simulink model "V1"  (R2025a)
settings: Solver=VariableStepAuto  StartTime=0.0  StopTime=200  FixedStep=0.005  RelTol=1e-3
libraries: cstblocks x11, vrlib x10, slpidlib x9, simulink_extras x8, dspinverses x3, robotcorelib x2, simulink x1
(part 2 of 3)

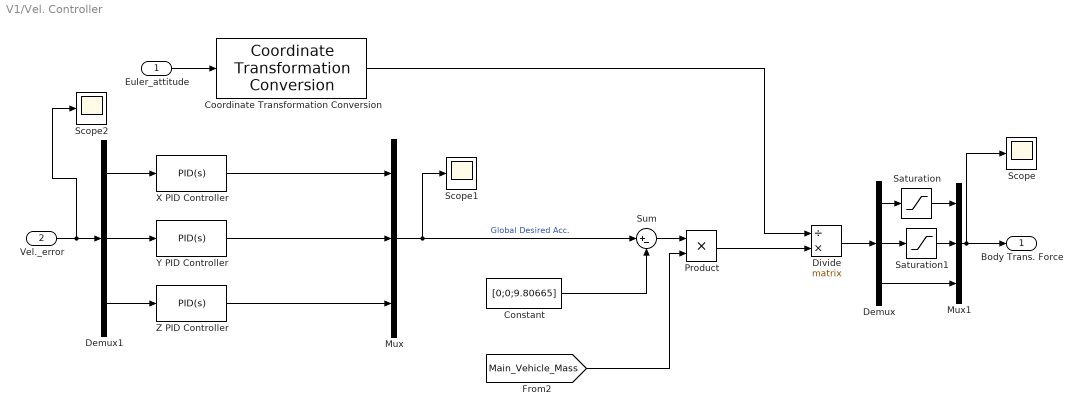
== system V1/Vel. Controller ==
  Euler_attitude : Inport
  Vel._error : Inport  Port=2
  Constant : Constant  Value=[0;0;9.80665]
  Coordinate Transformation Conversion : robotcorelib/Coordinate Transformation Conversion  InputRepresentation=Euler Angles  InputEulerSequence=XYZ  ShowTrVecInputPort=on  OutputRepresentation=Rotation Matrix  OutputEulerSequence=ZYX  ShowTrVecOutputPort=on  SimulateUsing=Interpreted execution
  Demux : Demux  Outputs=3
  Demux1 : Demux  Outputs=3
  Divide : Product  Inputs=/*  Multiplication=Matrix(*)
  Mux : Mux  Inputs=3
  Mux1 : Mux  Inputs=3
  Product : Product
  Saturation : Saturate  UpperLimit=50  LowerLimit=-50
  Saturation1 : Saturate  UpperLimit=50  LowerLimit=-50
  Scope : Scope
      settings: ActiveDisplayYMinimum=-41.94402  ActiveDisplayYMaximum=31.3207  DataLoggingVariableName=ScopeData2
  Scope1 : Scope
      settings: ActiveDisplayYMinimum=-15.22848  ActiveDisplayYMaximum=13.36333
  Scope2 : Scope
      settings: ActiveDisplayYMinimum=-406.2264  ActiveDisplayYMaximum=117.71416  DataLoggingVariableName=ScopeData4
  Sum : Sum  Inputs=|+-
  X PID Controller : slpidlib/PID Controller  Controller=PID  Form=Parallel  TimeDomain=Continuous-time  UseExternalTs=off  SampleTime=-1  IntegratorMethod=Forward Euler  FilterMethod=Forward Euler  ControllerParametersSource=internal  P=3  I=0  UseKiTs=off  D=1  UseExternalDerivativeSource=off  N=100  UseFilter=on  TunerSelectOption=Transfer Function Based (PID Tuner App)  InitialConditionSource=internal  InitialConditionForIntegrator=0  InitialConditionForFilter=0  DifferentiatorICPrevScaledInput=0  ExternalReset=none  TrackingMode=off  Kt=1  LimitOutput=off  SatLimitsSource=internal  UpperSaturationLimit=2  LowerSaturationLimit=-2  LinearizeAsGain=on  AntiWindupMode=none  Kb=1  LimitIntegrator=off  UpperIntegratorSaturationLimit=inf  LowerIntegratorSaturationLimit=-inf  POutMin=[]  POutMax=[]  IOutMin=[]  IOutMax=[]  DOutMin=[]  DOutMax=[]  NOutMin=[]  NOutMax=[]  SumOutMin=[]  SumOutMax=[]  SaturationOutMin=[]  SaturationOutMax=[]  PParamMin=[]  PParamMax=[]  IParamMin=[]  IParamMax=[]  DParamMin=[]  DParamMax=[]  NParamMin=[]  NParamMax=[]  KbParamMin=[]  KbParamMax=[]  KtParamMin=[]  KtParamMax=[]  KbOutMin=[]  KbOutMax=[]  KtOutMin=[]  KtOutMax=[]  IntegratorOutMin=[]  IntegratorOutMax=[]  FilterOutMin=[]  FilterOutMax=[]  SumI1OutMin=[]  SumI1OutMax=[]  SumI2OutMin=[]  SumI2OutMax=[]  SumI3OutMin=[]  SumI3OutMax=[]  SumI4OutMin=[]  SumI4OutMax=[]  SumDOutMin=[]  SumDOutMax=[]  DifferentiatorOutMin=[]  DifferentiatorOutMax=[]  FilterDiffOutCoefMin=[]  FilterDiffOutCoefMax=[]  ReciprocalOutMin=[]  ReciprocalOutMax=[]  SumDenOutMin=[]  SumDenOutMax=[]  SumNumOutMin=[]  SumNumOutMax=[]  DivideOutMin=[]  DivideOutMax=[]  UdiffTsProdOutMin=[]  UdiffTsProdOutMax=[]  NTsProdOutMin=[]  NTsProdOutMax=[]  UintegralTsProdOutMin=[]  UintegralTsProdOutMax=[]  UngainTsProdOutMin=[]  UngainTsProdOutMax=[]  ClampingZeroOutDataTypeStr=Inherit: Inherit via back propagation  ClampingZeroOutMin=[]  ClampingZeroOutMax=[]  FilterDenConstantOutDataTypeStr=Inherit: Inherit via back propagation  FilterDenConstantOutMin=[]  FilterDenConstantOutMax=[]  PCopyOutDataTypeStr=Inherit: Inherit via back propagation  PCopyOutMin=[]  PCopyOutMax=[]  NCopyOutDataTypeStr=Inherit: Inherit via back propagation  NCopyOutMin=[]  NCopyOutMax=[]  IntegratorContinuousStateAttributes=''  IntegratorStateMustResolveToSignalObject=off  IntegratorRTWStateStorageClass=Auto  FilterContinuousStateAttributes=''  FilterStateMustResolveToSignalObject=off  FilterRTWStateStorageClass=Auto  ParallelPVariant=InternalParameters  IdealPVariant=Disabled  IVariant=InternalParameters  DVariant=InternalParameters  IntegratorVariant=Continuous  SatVariant=Disabled  AWVariant=Passthrough  PCopyVariant=Disabled  TRVariant=Disabled  FdbkBlocksVariant=Forward  IdealPFdbkVariant=Disabled  SatFdbkVariant=Disabled  DerivativeFilterVariant=ContFilter  NVariant=InternalParameters  NCopyVariant=Disabled  FilterICVariant=InternalICsFilter  IntegratorICVariant=InternalICs  ExternalResetVariant=Disabled  TRSumVariant=Passthrough  SumFdbkVariant=Disabled  SumVariant=Sum_PID  TsampFilterVariant=InternalTs  TsampNgainVariant=Passthrough  TsampIntegralVariant=Disabled_SignalSpec  ExternalSaturationOutDataTypeStr=Inherit: Same as second input  DerivativeSourceVariant=ErrorSignal  PreIntVariant=InternalPreInt
  Y PID Controller : slpidlib/PID Controller  Controller=PID  Form=Parallel  TimeDomain=Continuous-time  UseExternalTs=off  SampleTime=-1  IntegratorMethod=Forward Euler  FilterMethod=Forward Euler  ControllerParametersSource=internal  P=3  I=0  UseKiTs=off  D=1  UseExternalDerivativeSource=off  N=100  UseFilter=on  TunerSelectOption=Transfer Function Based (PID Tuner App)  InitialConditionSource=internal  InitialConditionForIntegrator=0  InitialConditionForFilter=0  DifferentiatorICPrevScaledInput=0  ExternalReset=none  TrackingMode=off  Kt=1  LimitOutput=off  SatLimitsSource=internal  UpperSaturationLimit=2  LowerSaturationLimit=-2  LinearizeAsGain=on  AntiWindupMode=none  Kb=1  LimitIntegrator=off  UpperIntegratorSaturationLimit=inf  LowerIntegratorSaturationLimit=-inf  POutMin=[]  POutMax=[]  IOutMin=[]  IOutMax=[]  DOutMin=[]  DOutMax=[]  NOutMin=[]  NOutMax=[]  SumOutMin=[]  SumOutMax=[]  SaturationOutMin=[]  SaturationOutMax=[]  PParamMin=[]  PParamMax=[]  IParamMin=[]  IParamMax=[]  DParamMin=[]  DParamMax=[]  NParamMin=[]  NParamMax=[]  KbParamMin=[]  KbParamMax=[]  KtParamMin=[]  KtParamMax=[]  KbOutMin=[]  KbOutMax=[]  KtOutMin=[]  KtOutMax=[]  IntegratorOutMin=[]  IntegratorOutMax=[]  FilterOutMin=[]  FilterOutMax=[]  SumI1OutMin=[]  SumI1OutMax=[]  SumI2OutMin=[]  SumI2OutMax=[]  SumI3OutMin=[]  SumI3OutMax=[]  SumI4OutMin=[]  SumI4OutMax=[]  SumDOutMin=[]  SumDOutMax=[]  DifferentiatorOutMin=[]  DifferentiatorOutMax=[]  FilterDiffOutCoefMin=[]  FilterDiffOutCoefMax=[]  ReciprocalOutMin=[]  ReciprocalOutMax=[]  SumDenOutMin=[]  SumDenOutMax=[]  SumNumOutMin=[]  SumNumOutMax=[]  DivideOutMin=[]  DivideOutMax=[]  UdiffTsProdOutMin=[]  UdiffTsProdOutMax=[]  NTsProdOutMin=[]  NTsProdOutMax=[]  UintegralTsProdOutMin=[]  UintegralTsProdOutMax=[]  UngainTsProdOutMin=[]  UngainTsProdOutMax=[]  ClampingZeroOutDataTypeStr=Inherit: Inherit via back propagation  ClampingZeroOutMin=[]  ClampingZeroOutMax=[]  FilterDenConstantOutDataTypeStr=Inherit: Inherit via back propagation  FilterDenConstantOutMin=[]  FilterDenConstantOutMax=[]  PCopyOutDataTypeStr=Inherit: Inherit via back propagation  PCopyOutMin=[]  PCopyOutMax=[]  NCopyOutDataTypeStr=Inherit: Inherit via back propagation  NCopyOutMin=[]  NCopyOutMax=[]  IntegratorContinuousStateAttributes=''  IntegratorStateMustResolveToSignalObject=off  IntegratorRTWStateStorageClass=Auto  FilterContinuousStateAttributes=''  FilterStateMustResolveToSignalObject=off  FilterRTWStateStorageClass=Auto  ParallelPVariant=InternalParameters  IdealPVariant=Disabled  IVariant=InternalParameters  DVariant=InternalParameters  IntegratorVariant=Continuous  SatVariant=Disabled  AWVariant=Passthrough  PCopyVariant=Disabled  TRVariant=Disabled  FdbkBlocksVariant=Forward  IdealPFdbkVariant=Disabled  SatFdbkVariant=Disabled  DerivativeFilterVariant=ContFilter  NVariant=InternalParameters  NCopyVariant=Disabled  FilterICVariant=InternalICsFilter  IntegratorICVariant=InternalICs  ExternalResetVariant=Disabled  TRSumVariant=Passthrough  SumFdbkVariant=Disabled  SumVariant=Sum_PID  TsampFilterVariant=InternalTs  TsampNgainVariant=Passthrough  TsampIntegralVariant=Disabled_SignalSpec  ExternalSaturationOutDataTypeStr=Inherit: Same as second input  DerivativeSourceVariant=ErrorSignal  PreIntVariant=InternalPreInt
  Z PID Controller : slpidlib/PID Controller  Controller=PID  Form=Parallel  TimeDomain=Continuous-time  UseExternalTs=off  SampleTime=-1  IntegratorMethod=Forward Euler  FilterMethod=Forward Euler  ControllerParametersSource=internal  P=3  I=0  UseKiTs=off  D=1  UseExternalDerivativeSource=off  N=100  UseFilter=on  TunerSelectOption=Transfer Function Based (PID Tuner App)  InitialConditionSource=internal  InitialConditionForIntegrator=0  InitialConditionForFilter=0  DifferentiatorICPrevScaledInput=0  ExternalReset=none  TrackingMode=off  Kt=1  LimitOutput=off  SatLimitsSource=internal  UpperSaturationLimit=3  LowerSaturationLimit=-3  LinearizeAsGain=on  AntiWindupMode=none  Kb=1  LimitIntegrator=off  UpperIntegratorSaturationLimit=inf  LowerIntegratorSaturationLimit=-inf  POutMin=[]  POutMax=[]  IOutMin=[]  IOutMax=[]  DOutMin=[]  DOutMax=[]  NOutMin=[]  NOutMax=[]  SumOutMin=[]  SumOutMax=[]  SaturationOutMin=[]  SaturationOutMax=[]  PParamMin=[]  PParamMax=[]  IParamMin=[]  IParamMax=[]  DParamMin=[]  DParamMax=[]  NParamMin=[]  NParamMax=[]  KbParamMin=[]  KbParamMax=[]  KtParamMin=[]  KtParamMax=[]  KbOutMin=[]  KbOutMax=[]  KtOutMin=[]  KtOutMax=[]  IntegratorOutMin=[]  IntegratorOutMax=[]  FilterOutMin=[]  FilterOutMax=[]  SumI1OutMin=[]  SumI1OutMax=[]  SumI2OutMin=[]  SumI2OutMax=[]  SumI3OutMin=[]  SumI3OutMax=[]  SumI4OutMin=[]  SumI4OutMax=[]  SumDOutMin=[]  SumDOutMax=[]  DifferentiatorOutMin=[]  DifferentiatorOutMax=[]  FilterDiffOutCoefMin=[]  FilterDiffOutCoefMax=[]  ReciprocalOutMin=[]  ReciprocalOutMax=[]  SumDenOutMin=[]  SumDenOutMax=[]  SumNumOutMin=[]  SumNumOutMax=[]  DivideOutMin=[]  DivideOutMax=[]  UdiffTsProdOutMin=[]  UdiffTsProdOutMax=[]  NTsProdOutMin=[]  NTsProdOutMax=[]  UintegralTsProdOutMin=[]  UintegralTsProdOutMax=[]  UngainTsProdOutMin=[]  UngainTsProdOutMax=[]  ClampingZeroOutDataTypeStr=Inherit: Inherit via back propagation  ClampingZeroOutMin=[]  ClampingZeroOutMax=[]  FilterDenConstantOutDataTypeStr=Inherit: Inherit via back propagation  FilterDenConstantOutMin=[]  FilterDenConstantOutMax=[]  PCopyOutDataTypeStr=Inherit: Inherit via back propagation  PCopyOutMin=[]  PCopyOutMax=[]  NCopyOutDataTypeStr=Inherit: Inherit via back propagation  NCopyOutMin=[]  NCopyOutMax=[]  IntegratorContinuousStateAttributes=''  IntegratorStateMustResolveToSignalObject=off  IntegratorRTWStateStorageClass=Auto  FilterContinuousStateAttributes=''  FilterStateMustResolveToSignalObject=off  FilterRTWStateStorageClass=Auto  ParallelPVariant=InternalParameters  IdealPVariant=Disabled  IVariant=InternalParameters  DVariant=InternalParameters  IntegratorVariant=Continuous  SatVariant=Disabled  AWVariant=Passthrough  PCopyVariant=Disabled  TRVariant=Disabled  FdbkBlocksVariant=Forward  IdealPFdbkVariant=Disabled  SatFdbkVariant=Disabled  DerivativeFilterVariant=ContFilter  NVariant=InternalParameters  NCopyVariant=Disabled  FilterICVariant=InternalICsFilter  IntegratorICVariant=InternalICs  ExternalResetVariant=Disabled  TRSumVariant=Passthrough  SumFdbkVariant=Disabled  SumVariant=Sum_PID  TsampFilterVariant=InternalTs  TsampNgainVariant=Passthrough  TsampIntegralVariant=Disabled_SignalSpec  ExternalSaturationOutDataTypeStr=Inherit: Same as second input  DerivativeSourceVariant=ErrorSignal  PreIntVariant=InternalPreInt
  Body Trans. Force : Outport
  wires:
  X PID Controller/1 -> Mux/1
  Demux1/1 -> X PID Controller/1
  Demux1/3 -> Z PID Controller/1
  Demux1/2 -> Y PID Controller/1
  Y PID Controller/1 -> Mux/2
  Mux/1 -> Sum/1, Scope1/1  "Global Desired Acc."
  Z PID Controller/1 -> Mux/3
  Vel._error/1 -> Scope2/1, Demux1/1
  Constant/1 -> Sum/2
  Sum/1 -> Product/1
  Euler_attitude/1 -> Coordinate Transformation Conversion/1
  Coordinate Transformation Conversion/1 -> Divide/1
  [Main_Vehicle_Mass] -> Product/2
  Product/1 -> Divide/2
  Divide/1 -> Demux/1
  Demux/3 -> Mux1/3
  Demux/1 -> Saturation/1
  Demux/2 -> Saturation1/1
  Mux1/1 -> Scope/1, Body Trans. Force/1
  Saturation/1 -> Mux1/1
  Saturation1/1 -> Mux1/2

== system V1/skew-symmetric ==
  In1 : Inport
  Constant16 : Constant  Value=0
  Constant17 : Constant  Value=0
  Constant18 : Constant  Value=0
  Demux2 : Demux  Outputs=3
  Display : Display
  Gain : Gain  Gain=-1
  Gain1 : Gain  Gain=-1
  Gain2 : Gain  Gain=-1
  Mux{13..15,17} (4 alike) : Mux  Inputs=3
  Reshape : Reshape  OutputDimensionality=Customize  OutputDimensions=[3,3]
  Transpose : Math  Operator=transpose
  Out1 : Outport
  wires:
  Constant17/1 -> Mux14/2
  Gain2/1 -> Mux15/1
  Mux13/1 -> Mux17/1
  Reshape/1 -> Transpose/1
  Demux2/3 -> Mux14/1, Gain/1  "fz"
  Demux2/2 -> Gain2/1, Mux13/3  "fy"
  Constant18/1 -> Mux15/3
  Gain1/1 -> Mux14/3
  Demux2/1 -> Mux15/2, Gain1/1  "fx"
  Mux17/1 -> Reshape/1
  Mux14/1 -> Mux17/2
  Transpose/1 -> Display/1, Out1/1
  Mux15/1 -> Mux17/3
  Constant16/1 -> Mux13/1
  Gain/1 -> Mux13/2
  In1/1 -> Demux2/1

== system V1/skew-symmetric1 ==
  Constant16 : Constant  Value=3
  Constant17 : Constant  Value=2
  Constant18 : Constant
  Display : Display
  Mux{13..15,17} (4 alike) : Mux  Inputs=3
  Reshape : Reshape  OutputDimensionality=Customize  OutputDimensions=[3,3]
  Transpose : Math  Operator=transpose
  Out1 : Outport
  wires:
  Constant17/1 -> Mux14/2
  ? -> Mux15/1
  Mux13/1 -> Mux17/1
  Reshape/1 -> Transpose/1
  Constant18/1 -> Mux15/3
  ? -> Mux14/3
  Mux17/1 -> Reshape/1
  Mux14/1 -> Mux17/2
  Transpose/1 -> Display/1, Out1/1
  Mux15/1 -> Mux17/3
  Constant16/1 -> Mux13/1
  ? -> Mux13/2

== system V1/Attitude Controller/Subsystem ==
  Constant : Constant
  M11 : Outport
  wires:
  Constant/1 -> M11/1

== system V1/Attitude Controller/Subsystem1 ==
  Constant : Constant  Value=0
  M12 : Outport
  wires:
  Constant/1 -> M12/1

== system V1/Attitude Controller/Subsystem10 ==
  Product : Product
  Trigonometric Function : Trigonometry  Operator=cos
  Trigonometric Function1 : Trigonometry  Operator=cos
  M33 : Outport
  wires:
  Trigonometric Function/1 -> Product/1
  [roll] -> Trigonometric Function1/1
  [pitch] -> Trigonometric Function/1
  Product/1 -> M33/1
  Trigonometric Function1/1 -> Product/2

== system V1/Attitude Controller/Subsystem2 ==
  Gain : Gain  Gain=-1
  Trigonometric Function : Trigonometry
  M13 : Outport
  wires:
  Trigonometric Function/1 -> Gain/1
  [pitch] -> Trigonometric Function/1
  Gain/1 -> M13/1

== system V1/Attitude Controller/Subsystem4 ==
  Constant : Constant  Value=0
  M21 : Outport
  wires:
  Constant/1 -> M21/1

== system V1/Attitude Controller/Subsystem5 ==
  Trigonometric Function : Trigonometry  Operator=cos
  M22 : Outport
  wires:
  [roll] -> Trigonometric Function/1
  Trigonometric Function/1 -> M22/1

== system V1/Attitude Controller/Subsystem6 ==
  Product : Product
  Trigonometric Function : Trigonometry  Operator=cos
  Trigonometric Function1 : Trigonometry
  M23 : Outport
  wires:
  [pitch] -> Trigonometric Function/1
  Trigonometric Function/1 -> Product/1
  [roll] -> Trigonometric Function1/1
  Trigonometric Function1/1 -> Product/2
  Product/1 -> M23/1

== system V1/Attitude Controller/Subsystem8 ==
  Constant : Constant  Value=0
  M31 : Outport
  wires:
  Constant/1 -> M31/1

== system V1/Attitude Controller/Subsystem9 ==
  Gain : Gain  Gain=-1
  Trigonometric Function : Trigonometry
  M32 : Outport
  wires:
  [roll] -> Trigonometric Function/1
  Trigonometric Function/1 -> Gain/1
  Gain/1 -> M32/1

== system V1/Attitude Controller/Yaw rotation matrix ==
  Demux : Demux  Outputs=3
  Display : Display
  Gain : Gain  Gain=-1
  Mux1 : Mux
  Reshape : Reshape  OutputDimensionality=Customize  OutputDimensions=[2,2]
  Trigonometric Function : Trigonometry  Operator=cos
  Trigonometric Function1 : Trigonometry
  Trigonometric Function2 : Trigonometry
  Trigonometric Function3 : Trigonometry  Operator=cos
  Out1 : Outport
  wires:
  Trigonometric Function3/1 -> Mux1/4
  [current_yaw] -> Trigonometric Function3/1, Trigonometric Function2/1, Trigonometric Function1/1, Trigonometric Function/1
  Trigonometric Function/1 -> Mux1/1
  Reshape/1 -> Out1/1, Display/1
  Mux1/1 -> Reshape/1
  Demux/3 -> [current_yaw]
  [Euler_attitude] -> Demux/1
  Trigonometric Function2/1 -> Gain/1
  Trigonometric Function1/1 -> Mux1/2
  Gain/1 -> Mux1/3

== system V1/Body Frame Torque//Force/Subsystem ==
  theta_1 : Inport
  F1 : Inport  Port=2
  Constant : Constant  Value=sqrt(2)
  Divide : Product  Inputs=*/
  Gain : Gain  Gain=-1
  Mux : Mux  Inputs=3
  Product : Product
  Product2 : Product
  Scope : Scope
      settings: ActiveDisplayYMinimum=-32.89337  ActiveDisplayYMaximum=8.61151  DataLoggingVariableName=ScopeData6
  Trigonometric Function : Trigonometry
  Trigonometric Function2 : Trigonometry  Operator=cos
  F1_vector : Outport
  wires:
  Product/1 -> Divide/1
  F1/1 -> Product/2, Product2/2
  Divide/1 -> Mux/2, Mux/1
  theta_1/1 -> Trigonometric Function2/1, Trigonometric Function/1
  Constant/1 -> Divide/2
  Trigonometric Function2/1 -> Product2/1
  Trigonometric Function/1 -> Product/1
  Product2/1 -> Gain/1
  Gain/1 -> Mux/3
  Mux/1 -> Scope/1, F1_vector/1  "F1_vector"

== system V1/Body Frame Torque//Force/Subsystem1 ==
  theta_2 : Inport
  F2 : Inport  Port=2
  Constant : Constant  Value=sqrt(2)
  Divide : Product  Inputs=*/
  Gain : Gain  Gain=-1
  Gain1 : Gain  Gain=-1
  Mux : Mux  Inputs=3
  Product : Product
  Product2 : Product
  Trigonometric Function : Trigonometry
  Trigonometric Function2 : Trigonometry  Operator=cos
  F2_vector : Outport
  wires:
  Product/1 -> Divide/1
  F2/1 -> Product/2, Product2/2
  Divide/1 -> Gain1/1, Mux/1
  theta_2/1 -> Trigonometric Function2/1, Trigonometric Function/1
  Constant/1 -> Divide/2
  Trigonometric Function2/1 -> Product2/1
  Trigonometric Function/1 -> Product/1
  Product2/1 -> Gain/1
  Gain/1 -> Mux/3
  Mux/1 -> F2_vector/1  "F2_vector"
  Gain1/1 -> Mux/2

== system V1/Body Frame Torque//Force/Subsystem2 ==
  theta_3 : Inport
  F3 : Inport  Port=2
  Constant : Constant  Value=sqrt(2)
  Divide : Product  Inputs=*/
  Gain : Gain  Gain=-1
  Gain1 : Gain  Gain=-1
  Mux : Mux  Inputs=3
  Product : Product
  Product2 : Product
  Trigonometric Function : Trigonometry
  Trigonometric Function2 : Trigonometry  Operator=cos
  F3_vector : Outport
  wires:
  Product/1 -> Divide/1
  F3/1 -> Product/2, Product2/2
  theta_3/1 -> Trigonometric Function2/1, Trigonometric Function/1
  Constant/1 -> Divide/2
  Trigonometric Function2/1 -> Product2/1
  Trigonometric Function/1 -> Product/1
  Product2/1 -> Gain/1
  Gain/1 -> Mux/3
  Mux/1 -> F3_vector/1  "F3_vector"
  Divide/1 -> Gain1/1
  Gain1/1 -> Mux/2, Mux/1

== system V1/Body Frame Torque//Force/Subsystem3 ==
  theta_4 : Inport
  F4 : Inport  Port=2
  Constant : Constant  Value=sqrt(2)
  Divide : Product  Inputs=*/
  Gain : Gain  Gain=-1
  Gain1 : Gain  Gain=-1
  Mux : Mux  Inputs=3
  Product : Product
  Product2 : Product
  Trigonometric Function : Trigonometry
  Trigonometric Function2 : Trigonometry  Operator=cos
  F4_vector : Outport
  wires:
  Product/1 -> Divide/1
  F4/1 -> Product/2, Product2/2
  theta_4/1 -> Trigonometric Function2/1, Trigonometric Function/1
  Constant/1 -> Divide/2
  Trigonometric Function2/1 -> Product2/1
  Trigonometric Function/1 -> Product/1
  Product2/1 -> Gain/1
  Gain/1 -> Mux/3
  Mux/1 -> F4_vector/1  "F4_vector"
  Divide/1 -> Mux/2, Gain1/1
  Gain1/1 -> Mux/1

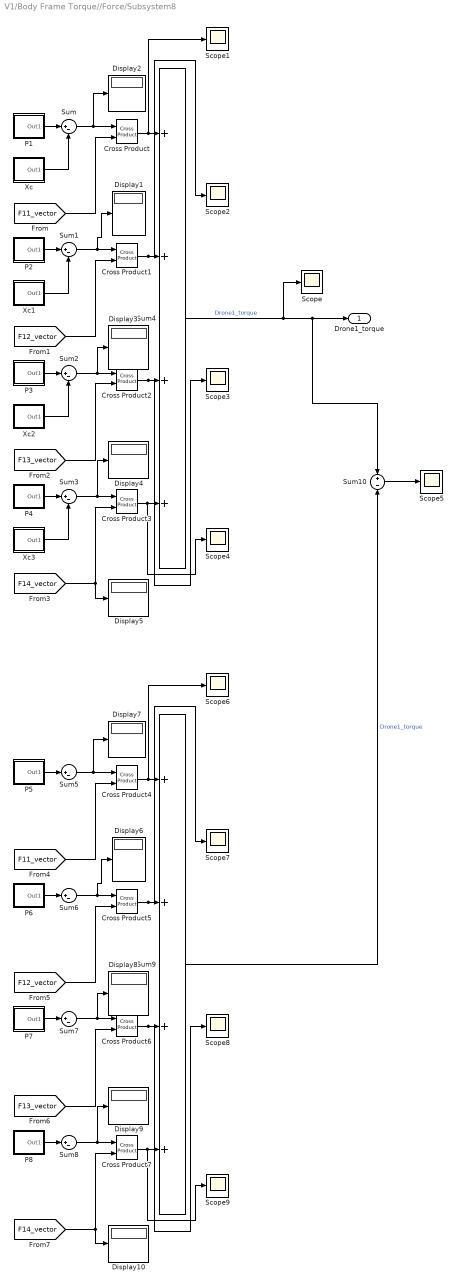
== system V1/Body Frame Torque//Force/Subsystem8 ==
  Cross Product{,1..7} (8 alike) : vrlib/Utilities/Cross Product
  Display{1..10} (10 alike) : Display
  P1 : Subsystem
  P2 : Subsystem
  P3 : Subsystem
  P4 : Subsystem
  P5 : Subsystem
  P6 : Subsystem
  P7 : Subsystem
  P8 : Subsystem
  Scope{,1..9} (10 alike) : Scope
      Scope settings: ActiveDisplayYMinimum=-18.62946  ActiveDisplayYMaximum=66.56889  DataLoggingVariableName=ScopeData4
      Scope1 settings: ActiveDisplayYMinimum=-10.54691  ActiveDisplayYMaximum=29.45294  DataLoggingVariableName=ScopeData10
      Scope2 settings: ActiveDisplayYMinimum=-40.74135  ActiveDisplayYMaximum=40.66911  DataLoggingVariableName=ScopeData11
      Scope3 settings: ActiveDisplayYMinimum=-10.03102  ActiveDisplayYMaximum=8.10812  DataLoggingVariableName=ScopeData15
      Scope4 settings: ActiveDisplayYMinimum=-1.76721  ActiveDisplayYMaximum=9.28155  DataLoggingVariableName=ScopeData16
      Scope5 settings: ActiveDisplayYMinimum=-2.09272  ActiveDisplayYMaximum=0.49282
      Scope6 settings: ActiveDisplayYMinimum=-10.73688  ActiveDisplayYMaximum=29.98451  DataLoggingVariableName=ScopeData2
      Scope7 settings: ActiveDisplayYMinimum=-56.63794  ActiveDisplayYMaximum=56.46415  DataLoggingVariableName=ScopeData3
      Scope8 settings: ActiveDisplayYMinimum=-10.03102  ActiveDisplayYMaximum=8.10812  DataLoggingVariableName=ScopeData4
      Scope9 settings: ActiveDisplayYMinimum=-1.76721  ActiveDisplayYMaximum=9.28155  DataLoggingVariableName=ScopeData5
  Sum{,1..3,5..8} (8 alike) : Sum  Inputs=|+-
  Sum10 : Sum  Inputs=+|-
  Sum4 : Sum  Inputs=++++
  Sum9 : Sum  Inputs=++++
  Xc : Subsystem
  Xc1 : Subsystem
  Xc2 : Subsystem
  Xc3 : Subsystem
  Drone1_torque : Outport
  wires:
  Xc3/1(Out1) -> Sum3/2
  Xc2/1(Out1) -> Sum2/2
  P4/1(Out1) -> Sum3/1
  [F11_vector] -> Cross Product/2
  [F12_vector] -> Cross Product1/2
  P3/1(Out1) -> Sum2/1
  Sum1/1 -> Cross Product1/1, Display1/1
  Cross Product1/1 -> Scope2/1, Sum4/2
  Xc/1(Out1) -> Sum/2
  [F14_vector] -> Cross Product3/2, Display5/1
  Sum/1 -> Display2/1, Cross Product/1
  P1/1(Out1) -> Sum/1
  Cross Product/1 -> Scope1/1, Sum4/1
  Xc1/1(Out1) -> Sum1/2
  Sum3/1 -> Display4/1, Cross Product3/1
  Sum2/1 -> Cross Product2/1, Display3/1
  [F13_vector] -> Cross Product2/2
  Cross Product2/1 -> Scope3/1, Sum4/3
  Cross Product3/1 -> Scope4/1, Sum4/4
  P2/1(Out1) -> Sum1/1
  Sum4/1 -> Scope/1, Sum10/1, Drone1_torque/1  "Drone1_torque"
  P8/1(Out1) -> Sum8/1
  Cross Product4/1 -> Scope6/1, Sum9/1
  Cross Product6/1 -> Scope8/1, Sum9/3
  Sum6/1 -> Cross Product5/1, Display6/1
  P6/1(Out1) -> Sum6/1
  P5/1(Out1) -> Sum5/1
  Cross Product7/1 -> Scope9/1, Sum9/4
  Cross Product5/1 -> Scope7/1, Sum9/2
  Sum5/1 -> Display7/1, Cross Product4/1
  [F13_vector] -> Cross Product6/2
  ? -> Sum5/2
  Sum7/1 -> Cross Product6/1, Display8/1
  [F11_vector] -> Cross Product4/2
  ? -> Sum6/2
  Sum8/1 -> Display9/1, Cross Product7/1
  [F14_vector] -> Cross Product7/2, Display10/1
  [F12_vector] -> Cross Product5/2
  ? -> Sum8/2
  Sum9/1 -> Sum10/2  "Drone1_torque"
  P7/1(Out1) -> Sum7/1
  ? -> Sum7/2
  Sum10/1 -> Scope5/1

== system V1/Non-sequential mixer/Wrench allocation_Drone1 ==
  In1 : Inport
  Bus Selector : BusSelector  OutputSignals=F_x,F_y,F_z
  Bus Selector2 : BusSelector  OutputSignals=tau_x,tau_y,tau_z
  Mux10 : Mux  Inputs=2
  Mux8 : Mux  Inputs=3
  Mux9 : Mux  Inputs=3
  Out1 : Outport
  wires:
  Bus Selector/2 -> Mux8/2  "<F_y>"
  Mux8/1 -> Mux10/2
  In1/1 -> Bus Selector/1, Bus Selector2/1
  Bus Selector2/3 -> Mux9/3  "<tau_z>"
  Bus Selector2/2 -> Mux9/2  "<tau_y>"
  Mux9/1 -> Mux10/1
  Bus Selector2/1 -> Mux9/1  "<tau_x>"
  Mux10/1 -> Out1/1
  Bus Selector/1 -> Mux8/1  "<F_x>"
  Bus Selector/3 -> Mux8/3  "<F_z>"

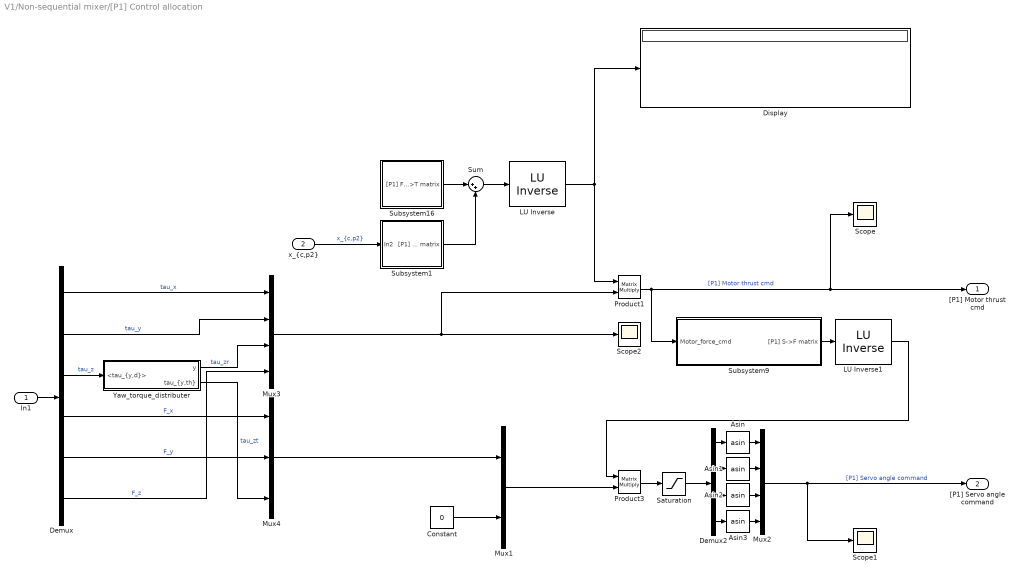
== system V1/Non-sequential mixer/[P1] Control allocation ==
  In1 : Inport
  "x_{c,p2}" : Inport  Port=2
  " LU Inverse" : dspinverses/ LU Inverse
  " LU Inverse1" : dspinverses/ LU Inverse
  Asin{,1..3} (4 alike) : Trigonometry  Operator=asin  OutputSignalType=real
  Constant : Constant  Value=0
  Demux : Demux  Outputs=6
  Demux2 : Demux
  Display : Display
  Mux1 : Mux  Inputs=2
  Mux2 : Mux
  Mux3 : Mux
  Mux4 : Mux  Inputs=3
  Product1 : Product  Multiplication=Matrix(*)
  Product3 : Product  Multiplication=Matrix(*)
  Saturation : Saturate  UpperLimit=0.9  LowerLimit=-0.9
  Scope : Scope
      settings: ActiveDisplayYMinimum=9.1632  ActiveDisplayYMaximum=24.163  DataLoggingVariableName=ScopeData3
  Scope1 : Scope
      settings: ActiveDisplayYMinimum=-1.39971  ActiveDisplayYMaximum=1.39971  DataLoggingVariableName=ScopeData4
  Scope2 : Scope
      settings: ActiveDisplayYMinimum=-7820.2372  ActiveDisplayYMaximum=1813.73582  DataLoggingVariableName=ScopeData5
  Subsystem1 : Subsystem
  Subsystem16 : Subsystem
  Subsystem9 : Subsystem
  Sum : Sum  Inputs=|++
  Yaw_torque_distributer : Subsystem
  "[P1] Motor thrust cmd" : Outport
  "[P1] Servo angle command" : Outport  Port=2
  wires:
  Product3/1 -> Saturation/1
  Subsystem9/1("[P1] S->F matrix") -> " LU Inverse1"/1
  Sum/1 -> " LU Inverse"/1
  Demux2/2 -> Asin1/1
  Asin1/1 -> Mux2/2
  Product1/1 -> Scope/1, "[P1] Motor thrust cmd"/1, Subsystem9/1(Motor_force_cmd)  "[P1] Motor thrust cmd"
  Mux1/1 -> Product3/2
  Asin2/1 -> Mux2/3
  " LU Inverse"/1 -> Product1/1, Display/1
  Mux2/1 -> Scope1/1, "[P1] Servo angle command"/1  "[P1] Servo angle command"
  Asin/1 -> Mux2/1
  Demux2/3 -> Asin2/1
  Asin3/1 -> Mux2/4
  Demux2/1 -> Asin/1
  " LU Inverse1"/1 -> Product3/1
  Demux2/4 -> Asin3/1
  Saturation/1 -> Demux2/1
  In1/1 -> Demux/1
  Demux/3 -> Yaw_torque_distributer/1("<tau_{y,d}>")  "tau_z"
  Demux/1 -> Mux3/1  "tau_x"
  Demux/2 -> Mux3/2  "tau_y"
  Yaw_torque_distributer/1(y) -> Mux3/3  "tau_zr"
  Demux/6 -> Mux3/4  "F_z"
  Demux/4 -> Mux4/1  "F_x"
  Demux/5 -> Mux4/2  "F_y"
  Yaw_torque_distributer/2("tau_{y,th}") -> Mux4/3  "tau_zt"
  "x_{c,p2}"/1 -> Subsystem1/1(In2)  "x_{c,p2}"
  Subsystem16/1("[P1] F->T matrix") -> Sum/1
  Subsystem1/1("[P1] F->T matrix") -> Sum/2
  Mux3/1 -> Scope2/1, Product1/2
  Mux4/1 -> Mux1/1
  Constant/1 -> Mux1/2

== system V1/Body Frame Torque//Force/Subsystem8/P1 ==
  Gain : Gain  Gain=1/sqrt(2)
  Gain1 : Gain  Gain=-1
  Mux : Mux  Inputs=3
  Out1 : Outport
  wires:
  Gain1/1 -> Mux/2
  [a] -> Mux/3
  [l] -> Gain/1
  Gain/1 -> Gain1/1, Mux/1
  Mux/1 -> Out1/1

== system V1/Body Frame Torque//Force/Subsystem8/P2 ==
  Gain : Gain  Gain=1/sqrt(2)
  Gain1 : Gain  Gain=-1
  Gain2 : Gain  Gain=-1
  Mux : Mux  Inputs=3
  Out1 : Outport
  wires:
  Gain1/1 -> Mux/2
  [a] -> Mux/3
  [l] -> Gain/1
  Gain/1 -> Gain1/1, Gain2/1
  Mux/1 -> Out1/1
  Gain2/1 -> Mux/1

== system V1/Body Frame Torque//Force/Subsystem8/P3 ==
  Gain : Gain  Gain=1/sqrt(2)
  Gain1 : Gain  Gain=-1
  Mux : Mux  Inputs=3
  Out1 : Outport
  wires:
  Gain/1 -> Mux/2, Gain1/1
  [a] -> Mux/3
  [l] -> Gain/1
  Mux/1 -> Out1/1
  Gain1/1 -> Mux/1

== system V1/Body Frame Torque//Force/Subsystem8/P4 ==
  Gain : Gain  Gain=1/sqrt(2)
  Mux : Mux  Inputs=3
  Out1 : Outport
  wires:
  Gain/1 -> Mux/2, Mux/1
  [a] -> Mux/3
  [l] -> Gain/1
  Mux/1 -> Out1/1

== system V1/Body Frame Torque//Force/Subsystem8/P5 ==
  Gain : Gain  Gain=1/sqrt(2)
  Gain1 : Gain  Gain=-1
  Mux : Mux  Inputs=3
  Out1 : Outport
  wires:
  Gain1/1 -> Mux/2
  [a] -> Mux/3
  [l] -> Gain/1
  Gain/1 -> Gain1/1, Mux/1
  Mux/1 -> Out1/1

== system V1/Body Frame Torque//Force/Subsystem8/P6 ==
  Gain : Gain  Gain=1/sqrt(2)
  Gain1 : Gain  Gain=-1
  Gain2 : Gain  Gain=-1
  Mux : Mux  Inputs=3
  Out1 : Outport
  wires:
  Gain1/1 -> Mux/2
  [a] -> Mux/3
  [l] -> Gain/1
  Gain/1 -> Gain1/1, Gain2/1
  Mux/1 -> Out1/1
  Gain2/1 -> Mux/1

== system V1/Body Frame Torque//Force/Subsystem8/P7 ==
  Gain : Gain  Gain=1/sqrt(2)
  Gain1 : Gain  Gain=-1
  Mux : Mux  Inputs=3
  Out1 : Outport
  wires:
  Gain/1 -> Mux/2, Gain1/1
  [a] -> Mux/3
  [l] -> Gain/1
  Mux/1 -> Out1/1
  Gain1/1 -> Mux/1

== system V1/Body Frame Torque//Force/Subsystem8/P8 ==
  Gain : Gain  Gain=1/sqrt(2)
  Mux : Mux  Inputs=3
  Out1 : Outport
  wires:
  Gain/1 -> Mux/2, Mux/1
  [a] -> Mux/3
  [l] -> Gain/1
  Mux/1 -> Out1/1

== system V1/Body Frame Torque//Force/Subsystem8/Xc ==
  Mux : Mux  Inputs=3
  Out1 : Outport
  wires:
  [x_c] -> Mux/1
  [z_c] -> Mux/3
  Mux/1 -> Out1/1
  [y_c] -> Mux/2

== system V1/Body Frame Torque//Force/Subsystem8/Xc1 ==
  Mux : Mux  Inputs=3
  Out1 : Outport
  wires:
  [x_c] -> Mux/1
  [z_c] -> Mux/3
  Mux/1 -> Out1/1
  [y_c] -> Mux/2

== system V1/Body Frame Torque//Force/Subsystem8/Xc2 ==
  Mux : Mux  Inputs=3
  Out1 : Outport
  wires:
  [x_c] -> Mux/1
  [z_c] -> Mux/3
  Mux/1 -> Out1/1
  [y_c] -> Mux/2

== system V1/Body Frame Torque//Force/Subsystem8/Xc3 ==
  Mux : Mux  Inputs=3
  Out1 : Outport
  wires:
  [x_c] -> Mux/1
  [z_c] -> Mux/3
  Mux/1 -> Out1/1
  [y_c] -> Mux/2

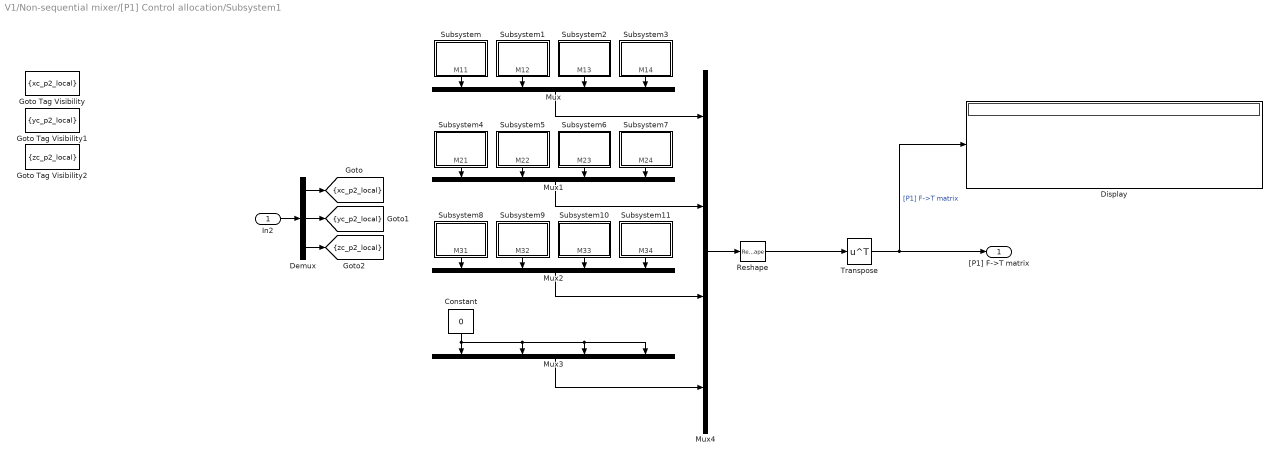
== system V1/Non-sequential mixer/[P1] Control allocation/Subsystem1 ==
  In2 : Inport
  Constant : Constant  Value=0
  Demux : Demux  Outputs=3
  Display : Display
  Goto Tag Visibility : GotoTagVisibility  GotoTag=xc_p2_local
  Goto Tag Visibility1 : GotoTagVisibility  GotoTag=yc_p2_local
  Goto Tag Visibility2 : GotoTagVisibility  GotoTag=zc_p2_local
  Mux{,1..4} (5 alike) : Mux
  Reshape : Reshape  OutputDimensionality=Customize  OutputDimensions=[4,4]
  Subsystem : Subsystem
  Subsystem1 : Subsystem
  Subsystem10 : Subsystem
  Subsystem11 : Subsystem
  Subsystem2 : Subsystem
  Subsystem3 : Subsystem
  Subsystem4 : Subsystem
  Subsystem5 : Subsystem
  Subsystem6 : Subsystem
  Subsystem7 : Subsystem
  Subsystem8 : Subsystem
  Subsystem9 : Subsystem
  Transpose : Math  Operator=transpose
  "[P1] F->T matrix" : Outport
  tag scope: xc_p2_local=scoped, yc_p2_local=scoped, zc_p2_local=scoped
  wires:
  Subsystem2/1(M13) -> Mux/3
  Constant/1 -> Mux3/4, Mux3/3, Mux3/2, Mux3/1
  Mux4/1 -> Reshape/1
  Subsystem8/1(M31) -> Mux2/1
  Mux3/1 -> Mux4/4
  Subsystem1/1(M12) -> Mux/2
  Subsystem5/1(M22) -> Mux1/2
  Subsystem11/1(M34) -> Mux2/4
  Subsystem7/1(M24) -> Mux1/4
  Reshape/1 -> Transpose/1
  Mux/1 -> Mux4/1
  Subsystem10/1(M33) -> Mux2/3
  Mux2/1 -> Mux4/3
  Subsystem3/1(M14) -> Mux/4
  Subsystem4/1(M21) -> Mux1/1
  Subsystem6/1(M23) -> Mux1/3
  Subsystem9/1(M32) -> Mux2/2
  Mux1/1 -> Mux4/2
  Subsystem/1(M11) -> Mux/1
  Transpose/1 -> "[P1] F->T matrix"/1, Display/1  "[P1] F->T matrix"
  In2/1 -> Demux/1
  Demux/1 -> [xc_p2_local]
  Demux/3 -> [zc_p2_local]
  Demux/2 -> [yc_p2_local]

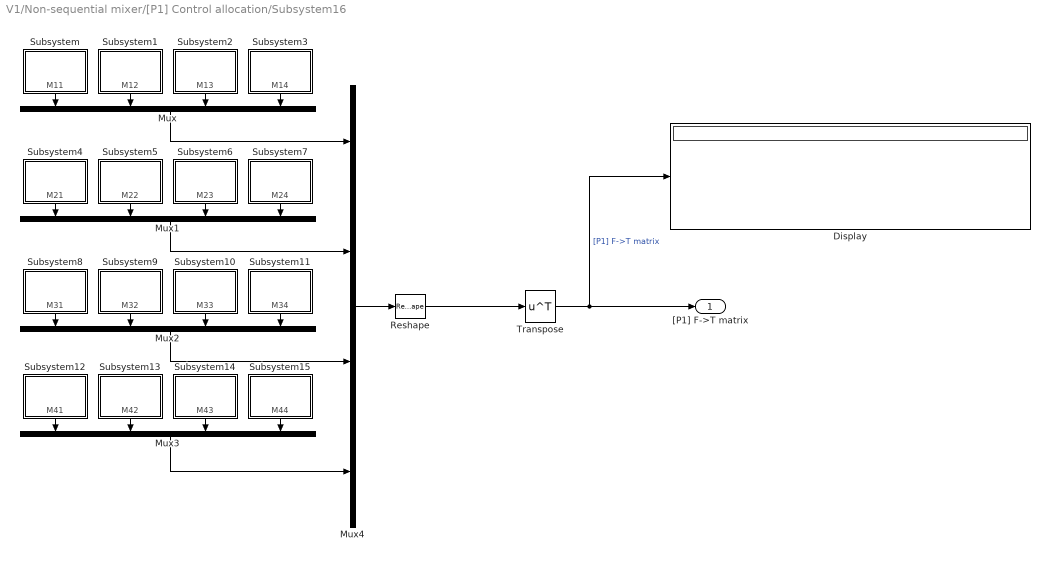
== system V1/Non-sequential mixer/[P1] Control allocation/Subsystem16 ==
  Display : Display
  Mux{,1..4} (5 alike) : Mux
  Reshape : Reshape  OutputDimensionality=Customize  OutputDimensions=[4,4]
  Subsystem : Subsystem
  Subsystem1 : Subsystem
  Subsystem10 : Subsystem
  Subsystem11 : Subsystem
  Subsystem12 : Subsystem
  Subsystem13 : Subsystem
  Subsystem14 : Subsystem
  Subsystem15 : Subsystem
  Subsystem2 : Subsystem
  Subsystem3 : Subsystem
  Subsystem4 : Subsystem
  Subsystem5 : Subsystem
  Subsystem6 : Subsystem
  Subsystem7 : Subsystem
  Subsystem8 : Subsystem
  Subsystem9 : Subsystem
  Transpose : Math  Operator=transpose
  "[P1] F->T matrix" : Outport
  wires:
  Subsystem2/1(M13) -> Mux/3
  Subsystem15/1(M44) -> Mux3/4
  Mux4/1 -> Reshape/1
  Subsystem8/1(M31) -> Mux2/1
  Subsystem14/1(M43) -> Mux3/3
  Mux3/1 -> Mux4/4
  Subsystem1/1(M12) -> Mux/2
  Subsystem5/1(M22) -> Mux1/2
  Subsystem11/1(M34) -> Mux2/4
  Subsystem7/1(M24) -> Mux1/4
  Reshape/1 -> Transpose/1
  Mux/1 -> Mux4/1
  Subsystem10/1(M33) -> Mux2/3
  Mux2/1 -> Mux4/3
  Subsystem3/1(M14) -> Mux/4
  Subsystem12/1(M41) -> Mux3/1
  Subsystem13/1(M42) -> Mux3/2
  Subsystem4/1(M21) -> Mux1/1
  Subsystem6/1(M23) -> Mux1/3
  Subsystem9/1(M32) -> Mux2/2
  Mux1/1 -> Mux4/2
  Subsystem/1(M11) -> Mux/1
  Transpose/1 -> "[P1] F->T matrix"/1, Display/1  "[P1] F->T matrix"

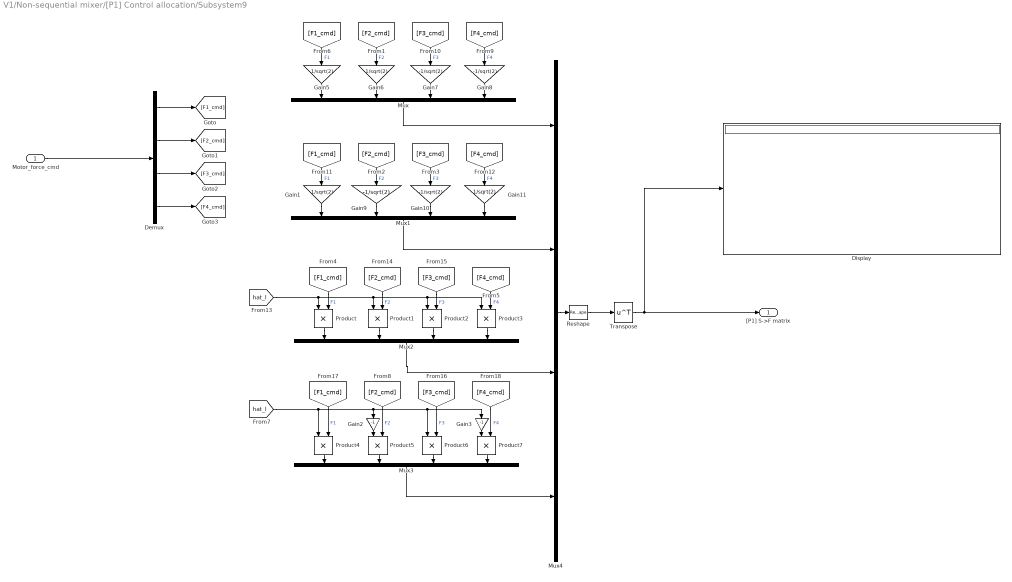
== system V1/Non-sequential mixer/[P1] Control allocation/Subsystem9 ==
  Motor_force_cmd : Inport
  Demux : Demux
  Display : Display
  Gain{1,5..6,11} (4 alike) : Gain  Gain=1/sqrt(2)
  Gain{7..10} (4 alike) : Gain  Gain=-1/sqrt(2)
  Gain2 : Gain  Gain=-1
  Gain3 : Gain  Gain=-1
  Mux{,1..4} (5 alike) : Mux
  Product{,1..7} (8 alike) : Product
  Reshape : Reshape  OutputDimensionality=Customize  OutputDimensions=[4,4]
  Transpose : Math  Operator=transpose
  "[P1] S->F matrix" : Outport
  wires:
  [F2_cmd] -> Gain6/1  "F2"
  Mux/1 -> Mux4/1
  Demux/2 -> [F2_cmd]
  [F1_cmd] -> Gain5/1  "F1"
  Demux/4 -> [F4_cmd]
  Mux3/1 -> Mux4/4
  Demux/3 -> [F3_cmd]
  Mux1/1 -> Mux4/2
  Mux2/1 -> Mux4/3
  Demux/1 -> [F1_cmd]
  Motor_force_cmd/1 -> Demux/1
  Mux4/1 -> Reshape/1
  Reshape/1 -> Transpose/1
  Transpose/1 -> "[P1] S->F matrix"/1, Display/1
  Gain5/1 -> Mux/1
  Gain6/1 -> Mux/2
  [F4_cmd] -> Gain8/1  "F4"
  [F3_cmd] -> Gain7/1  "F3"
  Gain7/1 -> Mux/3
  Gain8/1 -> Mux/4
  Gain9/1 -> Mux1/2
  Gain1/1 -> Mux1/1
  [F1_cmd] -> Gain1/1  "F1"
  [F2_cmd] -> Gain9/1  "F2"
  Gain11/1 -> Mux1/4
  Gain10/1 -> Mux1/3
  [F4_cmd] -> Gain11/1  "F4"
  [F3_cmd] -> Gain10/1  "F3"
  Product/1 -> Mux2/1
  Product1/1 -> Mux2/2
  Product2/1 -> Mux2/3
  Product3/1 -> Mux2/4
  [hat_l] -> Product3/1, Product2/1, Product1/1, Product/1
  [F1_cmd] -> Product/2  "F1"
  [F2_cmd] -> Product1/2  "F2"
  [F3_cmd] -> Product2/2  "F3"
  [F4_cmd] -> Product3/2  "F4"
  [hat_l] -> Gain3/1, Product6/1, Gain2/1, Product4/1
  [F4_cmd] -> Product7/2  "F4"
  Product5/1 -> Mux3/2
  Product4/1 -> Mux3/1
  Product7/1 -> Mux3/4
  [F2_cmd] -> Product5/2  "F2"
  Product6/1 -> Mux3/3
  [F3_cmd] -> Product6/2  "F3"
  [F1_cmd] -> Product4/2  "F1"
  Gain2/1 -> Product5/1
  Gain3/1 -> Product7/1

== system V1/Non-sequential mixer/[P1] Control allocation/Yaw_torque_distributer ==
  "<tau_{y,d}>" : Inport
  Gain : Gain  Gain=-1
  LTI System : cstblocks/LTI System  sys=tf(1,[1 10])  IC=[]  PadeOrder=0
  Saturation Dynamic : simulink/Discontinuities/Saturation Dynamic  OutMin=[]  OutMax=[]  OutDataTypeStr=Inherit: Same as second input  OutDataType=fixdt(1, 16)  OutScaling=2^-10  DoSatur=off
  Scope : Scope  NumInputPorts=2
      settings: ActiveDisplayYMinimum=-0.98774  ActiveDisplayYMaximum=2.13909
  Sum : Sum  Inputs=+-|
  Sum1 : Sum  Inputs=|+-
  Sum2 : Sum  Inputs=++|
  y : Outport
  "tau_{y,th}" : Outport  Port=2
  wires:
  Saturation Dynamic/1 -> Sum/2, Scope/1, y/1
  [yaw_torque_limit] -> Gain/1, Saturation Dynamic/1
  "<tau_{y,d}>"/1 -> Sum1/1, LTI System/1
  Gain/1 -> Saturation Dynamic/3
  LTI System/1 -> Sum1/2, Sum2/2
  Sum1/1 -> Sum/1, Saturation Dynamic/2  "tau_{y,th}"
  Sum/1 -> Sum2/1  "tau_{y,th}"
  Sum2/1 -> Scope/2, "tau_{y,th}"/1  "tau_{y,th}"

== system V1/Non-sequential mixer/[P1] Control allocation/Subsystem1/Subsystem ==
  Bus Selector : BusSelector  OutputSignals=theta_1
  Bus Selector1 : BusSelector  OutputSignals=theta_1
  Gain2 : Gain  Gain=1/sqrt(2)
  Product : Product
  Product1 : Product
  Sum1 : Sum  Inputs=|++
  Trigonometric Function : Trigonometry  Operator=cos
  Trigonometric Function1 : Trigonometry
  M11 : Outport
  wires:
  Product/1 -> Sum1/1
  Trigonometric Function/1 -> Product/2
  Bus Selector/1 -> Trigonometric Function/1  "<theta_1>"
  [zc_p2_local] -> Product1/1
  Product1/1 -> Gain2/1
  Trigonometric Function1/1 -> Product1/2
  Bus Selector1/1 -> Trigonometric Function1/1  "<theta_1>"
  [Sensor] -> Bus Selector/1
  [Sensor] -> Bus Selector1/1
  Sum1/1 -> M11/1  "M11"
  [yc_p2_local] -> Product/1
  Gain2/1 -> Sum1/2

== system V1/Non-sequential mixer/[P1] Control allocation/Subsystem1/Subsystem1 ==
  Bus Selector : BusSelector  OutputSignals=theta_2
  Bus Selector1 : BusSelector  OutputSignals=theta_2
  Gain1 : Gain  Gain=1/sqrt(2)
  Product : Product
  Product1 : Product
  Sum1 : Sum  Inputs=|+-
  Trigonometric Function : Trigonometry  Operator=cos
  Trigonometric Function1 : Trigonometry
  M12 : Outport
  wires:
  Product/1 -> Sum1/1
  [yc_p2_local] -> Product/1
  Trigonometric Function/1 -> Product/2
  Bus Selector/1 -> Trigonometric Function/1  "<theta_2>"
  [zc_p2_local] -> Product1/1
  Product1/1 -> Gain1/1
  Trigonometric Function1/1 -> Product1/2
  Bus Selector1/1 -> Trigonometric Function1/1  "<theta_2>"
  [Sensor] -> Bus Selector/1
  [Sensor] -> Bus Selector1/1
  Sum1/1 -> M12/1  "M12"
  Gain1/1 -> Sum1/2

== system V1/Non-sequential mixer/[P1] Control allocation/Subsystem1/Subsystem10 ==
  Bus Selector : BusSelector  OutputSignals=theta_3
  Constant : Constant  Value=sqrt(2)
  Divide : Product  Inputs=*/
  Product2 : Product
  Sum : Sum  Inputs=|+-
  Trigonometric Function : Trigonometry
  M33 : Outport
  wires:
  Trigonometric Function/1 -> Product2/2
  Bus Selector/1 -> Trigonometric Function/1  "<theta_3>"
  Divide/1 -> M33/1
  Constant/1 -> Divide/2
  [yc_p2_local] -> Sum/2
  Product2/1 -> Divide/1
  [Sensor] -> Bus Selector/1
  [xc_p2_local] -> Sum/1
  Sum/1 -> Product2/1

== system V1/Non-sequential mixer/[P1] Control allocation/Subsystem1/Subsystem11 ==
  Bus Selector : BusSelector  OutputSignals=theta_4
  Constant : Constant  Value=-sqrt(2)
  Divide : Product  Inputs=*/
  Product2 : Product
  Sum : Sum  Inputs=|++
  Trigonometric Function : Trigonometry
  M34 : Outport
  wires:
  Divide/1 -> M34/1
  Sum/1 -> Product2/1
  [yc_p2_local] -> Sum/2
  [Sensor] -> Bus Selector/1
  Constant/1 -> Divide/2
  Product2/1 -> Divide/1
  Bus Selector/1 -> Trigonometric Function/1  "<theta_4>"
  Trigonometric Function/1 -> Product2/2
  [xc_p2_local] -> Sum/1

== system V1/Non-sequential mixer/[P1] Control allocation/Subsystem1/Subsystem2 ==
  Bus Selector : BusSelector  OutputSignals=theta_3
  Bus Selector1 : BusSelector  OutputSignals=theta_3
  Gain2 : Gain  Gain=1/sqrt(2)
  Product : Product
  Product1 : Product
  Sum1 : Sum  Inputs=|+-
  Trigonometric Function : Trigonometry  Operator=cos
  Trigonometric Function1 : Trigonometry
  M13 : Outport
  wires:
  Product/1 -> Sum1/1
  Trigonometric Function/1 -> Product/2
  Bus Selector/1 -> Trigonometric Function/1  "<theta_3>"
  [zc_p2_local] -> Product1/1
  Product1/1 -> Gain2/1
  Trigonometric Function1/1 -> Product1/2
  Bus Selector1/1 -> Trigonometric Function1/1  "<theta_3>"
  [Sensor] -> Bus Selector/1
  [Sensor] -> Bus Selector1/1
  Sum1/1 -> M13/1  "M13"
  [yc_p2_local] -> Product/1
  Gain2/1 -> Sum1/2

== system V1/Non-sequential mixer/[P1] Control allocation/Subsystem1/Subsystem3 ==
  Bus Selector : BusSelector  OutputSignals=theta_4
  Bus Selector1 : BusSelector  OutputSignals=theta_4
  Gain2 : Gain  Gain=1/sqrt(2)
  Product : Product
  Product1 : Product
  Sum1 : Sum  Inputs=|++
  Trigonometric Function : Trigonometry  Operator=cos
  Trigonometric Function1 : Trigonometry
  M14 : Outport
  wires:
  Product/1 -> Sum1/1
  Trigonometric Function/1 -> Product/2
  Bus Selector/1 -> Trigonometric Function/1  "<theta_4>"
  [zc_p2_local] -> Product1/1
  Product1/1 -> Gain2/1
  Trigonometric Function1/1 -> Product1/2
  Bus Selector1/1 -> Trigonometric Function1/1  "<theta_4>"
  [Sensor] -> Bus Selector/1
  [Sensor] -> Bus Selector1/1
  Sum1/1 -> M14/1  "M14"
  [yc_p2_local] -> Product/1
  Gain2/1 -> Sum1/2

== system V1/Non-sequential mixer/[P1] Control allocation/Subsystem1/Subsystem4 ==
  Bus Selector2 : BusSelector  OutputSignals=theta_1
  Bus Selector3 : BusSelector  OutputSignals=theta_1
  Gain3 : Gain  Gain=1/sqrt(2)
  Product2 : Product
  Product3 : Product
  Sum4 : Sum  Inputs=|--
  Trigonometric Function2 : Trigonometry  Operator=cos
  Trigonometric Function3 : Trigonometry
  M21 : Outport
  wires:
  Sum4/1 -> M21/1  "M21"
  [zc_p2_local] -> Product3/1
  Gain3/1 -> Sum4/2
  [xc_p2_local] -> Product2/1
  [Sensor] -> Bus Selector2/1
  [Sensor] -> Bus Selector3/1
  Trigonometric Function3/1 -> Product3/2
  Bus Selector2/1 -> Trigonometric Function2/1  "<theta_1>"
  Trigonometric Function2/1 -> Product2/2
  Product3/1 -> Gain3/1
  Product2/1 -> Sum4/1
  Bus Selector3/1 -> Trigonometric Function3/1  "<theta_1>"

== system V1/Non-sequential mixer/[P1] Control allocation/Subsystem1/Subsystem5 ==
  Bus Selector2 : BusSelector  OutputSignals=theta_2
  Bus Selector3 : BusSelector  OutputSignals=theta_2
  Gain2 : Gain  Gain=1/sqrt(2)
  Product2 : Product
  Product3 : Product
  Sum2 : Sum  Inputs=|--
  Trigonometric Function2 : Trigonometry  Operator=cos
  Trigonometric Function3 : Trigonometry
  M22 : Outport
  wires:
  [xc_p2_local] -> Product2/1
  Sum2/1 -> M22/1
  [Sensor] -> Bus Selector3/1
  [Sensor] -> Bus Selector2/1
  Bus Selector3/1 -> Trigonometric Function3/1  "<theta_2>"
  Trigonometric Function3/1 -> Product3/2
  Product2/1 -> Sum2/1
  Bus Selector2/1 -> Trigonometric Function2/1  "<theta_2>"
  Trigonometric Function2/1 -> Product2/2
  Product3/1 -> Gain2/1
  [zc_p2_local] -> Product3/1
  Gain2/1 -> Sum2/2

== system V1/Non-sequential mixer/[P1] Control allocation/Subsystem1/Subsystem6 ==
  Bus Selector : BusSelector  OutputSignals=theta_3
  Bus Selector1 : BusSelector  OutputSignals=theta_3
  Gain2 : Gain  Gain=1/sqrt(2)
  Product : Product
  Product1 : Product
  Sum1 : Sum  Inputs=|-+
  Trigonometric Function : Trigonometry  Operator=cos
  Trigonometric Function1 : Trigonometry
  M23 : Outport
  wires:
  [Sensor] -> Bus Selector/1
  Bus Selector1/1 -> Trigonometric Function1/1  "<theta_3>"
  Bus Selector/1 -> Trigonometric Function/1  "<theta_3>"
  Product1/1 -> Gain2/1
  Trigonometric Function/1 -> Product/2
  [Sensor] -> Bus Selector1/1
  [zc_p2_local] -> Product1/1
  Product/1 -> Sum1/1
  Trigonometric Function1/1 -> Product1/2
  Gain2/1 -> Sum1/2
  [xc_p2_local] -> Product/1
  Sum1/1 -> M23/1

== system V1/Non-sequential mixer/[P1] Control allocation/Subsystem1/Subsystem7 ==
  Bus Selector : BusSelector  OutputSignals=theta_4
  Bus Selector1 : BusSelector  OutputSignals=theta_4
  Gain2 : Gain  Gain=1/sqrt(2)
  Product : Product
  Product1 : Product
  Sum1 : Sum  Inputs=|-+
  Trigonometric Function : Trigonometry  Operator=cos
  Trigonometric Function1 : Trigonometry
  M24 : Outport
  wires:
  [zc_p2_local] -> Product1/1
  [xc_p2_local] -> Product/1
  [Sensor] -> Bus Selector1/1
  Sum1/1 -> M24/1  "M14"
  Bus Selector1/1 -> Trigonometric Function1/1  "<theta_4>"
  [Sensor] -> Bus Selector/1
  Trigonometric Function1/1 -> Product1/2
  Trigonometric Function/1 -> Product/2
  Product1/1 -> Gain2/1
  Gain2/1 -> Sum1/2
  Product/1 -> Sum1/1
  Bus Selector/1 -> Trigonometric Function/1  "<theta_4>"

== system V1/Non-sequential mixer/[P1] Control allocation/Subsystem1/Subsystem8 ==
  Bus Selector : BusSelector  OutputSignals=theta_1
  Constant : Constant  Value=-sqrt(2)
  Divide : Product  Inputs=*/
  Product2 : Product
  Sum : Sum  Inputs=|+-
  Trigonometric Function : Trigonometry
  M31 : Outport
  wires:
  Bus Selector/1 -> Trigonometric Function/1  "<theta_1>"
  [Sensor] -> Bus Selector/1
  Trigonometric Function/1 -> Product2/2
  Product2/1 -> Divide/1
  [xc_p2_local] -> Sum/1
  [yc_p2_local] -> Sum/2
  Sum/1 -> Product2/1
  Constant/1 -> Divide/2
  Divide/1 -> M31/1

== system V1/Non-sequential mixer/[P1] Control allocation/Subsystem1/Subsystem9 ==
  Bus Selector : BusSelector  OutputSignals=theta_2
  Constant : Constant  Value=sqrt(2)
  Divide : Product  Inputs=*/
  Product2 : Product
  Sum : Sum  Inputs=|++
  Trigonometric Function : Trigonometry
  M32 : Outport
  wires:
  Divide/1 -> M32/1
  [yc_p2_local] -> Sum/2
  Sum/1 -> Product2/1
  [Sensor] -> Bus Selector/1
  Product2/1 -> Divide/1
  Bus Selector/1 -> Trigonometric Function/1  "<theta_2>"
  Trigonometric Function/1 -> Product2/2
  Constant/1 -> Divide/2
  [xc_p2_local] -> Sum/1

== system V1/Non-sequential mixer/[P1] Control allocation/Subsystem16/Subsystem ==
  Bus Selector : BusSelector  OutputSignals=theta_1
  Bus Selector1 : BusSelector  OutputSignals=theta_1
  Gain : Gain  Gain=1/sqrt(2)
  Gain1 : Gain  Gain=1/sqrt(2)
  Product : Product
  Product1 : Product
  Sum : Sum  Inputs=|++
  Sum1 : Sum  Inputs=|++
  Sum2 : Sum  Inputs=|+-
  Sum3 : Sum  Inputs=|--
  Trigonometric Function : Trigonometry  Operator=cos
  Trigonometric Function1 : Trigonometry
  M11 : Outport
  wires:
  Product/1 -> Sum1/1
  Sum/1 -> Product/1
  Sum2/1 -> Sum3/1
  Trigonometric Function/1 -> Product/2
  Bus Selector/1 -> Trigonometric Function/1  "<theta_1>"
  [hat_a] -> Sum2/1
  Gain/1 -> Sum/2
  Sum3/1 -> Gain1/1
  [hat_b_over_k] -> Sum3/2
  Gain1/1 -> Product1/1
  [hat_l] -> Gain/1
  Product1/1 -> Sum1/2
  Trigonometric Function1/1 -> Product1/2
  Bus Selector1/1 -> Trigonometric Function1/1  "<theta_1>"
  [Sensor] -> Bus Selector/1
  [Sensor] -> Bus Selector1/1
  Sum1/1 -> M11/1  "M11"

== system V1/Non-sequential mixer/[P1] Control allocation/Subsystem16/Subsystem1 ==
  Bus Selector : BusSelector  OutputSignals=theta_2
  Bus Selector1 : BusSelector  OutputSignals=theta_2
  Gain : Gain  Gain=1/sqrt(2)
  Gain1 : Gain  Gain=1/sqrt(2)
  Product : Product
  Product1 : Product
  Sum : Sum  Inputs=|++
  Sum1 : Sum  Inputs=|++
  Sum2 : Sum  Inputs=|+-
  Sum3 : Sum  Inputs=|++
  Trigonometric Function : Trigonometry  Operator=cos
  Trigonometric Function1 : Trigonometry
  M12 : Outport
  wires:
  Product/1 -> Sum1/1
  Sum/1 -> Product/1
  Sum2/1 -> Sum3/1
  Trigonometric Function/1 -> Product/2
  Bus Selector/1 -> Trigonometric Function/1  "<theta_2>"
  [hat_a] -> Sum2/1
  Gain/1 -> Sum/2
  Sum3/1 -> Gain1/1
  [hat_b_over_k] -> Sum3/2
  Gain1/1 -> Product1/1
  [hat_l] -> Gain/1
  Product1/1 -> Sum1/2
  Trigonometric Function1/1 -> Product1/2
  Bus Selector1/1 -> Trigonometric Function1/1  "<theta_2>"
  [Sensor] -> Bus Selector/1
  [Sensor] -> Bus Selector1/1
  Sum1/1 -> M12/1  "M12"

== system V1/Non-sequential mixer/[P1] Control allocation/Subsystem16/Subsystem10 ==
  Bus Selector : BusSelector  OutputSignals=theta_3
  Product2 : Product
  Trigonometric Function : Trigonometry  Operator=cos
  M33 : Outport
  wires:
  Bus Selector/1 -> Trigonometric Function/1  "<theta_3>"
  [Sensor] -> Bus Selector/1
  Trigonometric Function/1 -> Product2/2
  [hat_b_over_k] -> Product2/1
  Product2/1 -> M33/1

== system V1/Non-sequential mixer/[P1] Control allocation/Subsystem16/Subsystem11 ==
  Bus Selector : BusSelector  OutputSignals=theta_4
  Gain : Gain  Gain=-1
  Product2 : Product
  Trigonometric Function : Trigonometry  Operator=cos
  M34 : Outport
  wires:
  Bus Selector/1 -> Trigonometric Function/1  "<theta_4>"
  [Sensor] -> Bus Selector/1
  Trigonometric Function/1 -> Product2/2
  [hat_b_over_k] -> Product2/1
  Product2/1 -> Gain/1
  Gain/1 -> M34/1

== system V1/Non-sequential mixer/[P1] Control allocation/Subsystem16/Subsystem12 ==
  Bus Selector : BusSelector  OutputSignals=theta_1
  Gain2 : Gain  Gain=-1
  Trigonometric Function : Trigonometry  Operator=cos
  M41 : Outport
  wires:
  Bus Selector/1 -> Trigonometric Function/1  "<theta_1>"
  [Sensor] -> Bus Selector/1
  Gain2/1 -> M41/1
  Trigonometric Function/1 -> Gain2/1

== system V1/Non-sequential mixer/[P1] Control allocation/Subsystem16/Subsystem13 ==
  Bus Selector : BusSelector  OutputSignals=theta_2
  Gain2 : Gain  Gain=-1
  Trigonometric Function : Trigonometry  Operator=cos
  M42 : Outport
  wires:
  Bus Selector/1 -> Trigonometric Function/1  "<theta_2>"
  [Sensor] -> Bus Selector/1
  Gain2/1 -> M42/1
  Trigonometric Function/1 -> Gain2/1

== system V1/Non-sequential mixer/[P1] Control allocation/Subsystem16/Subsystem14 ==
  Bus Selector : BusSelector  OutputSignals=theta_3
  Gain2 : Gain  Gain=-1
  Trigonometric Function : Trigonometry  Operator=cos
  M43 : Outport
  wires:
  Bus Selector/1 -> Trigonometric Function/1  "<theta_3>"
  [Sensor] -> Bus Selector/1
  Gain2/1 -> M43/1
  Trigonometric Function/1 -> Gain2/1

== system V1/Non-sequential mixer/[P1] Control allocation/Subsystem16/Subsystem15 ==
  Bus Selector : BusSelector  OutputSignals=theta_4
  Gain2 : Gain  Gain=-1
  Trigonometric Function : Trigonometry  Operator=cos
  M44 : Outport
  wires:
  Bus Selector/1 -> Trigonometric Function/1  "<theta_4>"
  [Sensor] -> Bus Selector/1
  Gain2/1 -> M44/1
  Trigonometric Function/1 -> Gain2/1

== system V1/Non-sequential mixer/[P1] Control allocation/Subsystem16/Subsystem2 ==
  Bus Selector : BusSelector  OutputSignals=theta_3
  Bus Selector1 : BusSelector  OutputSignals=theta_3
  Gain : Gain  Gain=1/sqrt(2)
  Gain1 : Gain  Gain=1/sqrt(2)
  Product : Product
  Product1 : Product
  Sum : Sum  Inputs=|+-
  Sum1 : Sum  Inputs=|++
  Sum2 : Sum  Inputs=|+-
  Sum3 : Sum  Inputs=|++
  Trigonometric Function : Trigonometry  Operator=cos
  Trigonometric Function1 : Trigonometry
  M13 : Outport
  wires:
  Product/1 -> Sum1/1
  Sum/1 -> Product/1
  Sum2/1 -> Sum3/1
  Trigonometric Function/1 -> Product/2
  Bus Selector/1 -> Trigonometric Function/1  "<theta_3>"
  [hat_a] -> Sum2/1
  Gain/1 -> Sum/2
  Sum3/1 -> Gain1/1
  [hat_b_over_k] -> Sum3/2
  Gain1/1 -> Product1/1
  [hat_l] -> Gain/1
  Product1/1 -> Sum1/2
  Trigonometric Function1/1 -> Product1/2
  Bus Selector1/1 -> Trigonometric Function1/1  "<theta_3>"
  [Sensor] -> Bus Selector/1
  [Sensor] -> Bus Selector1/1
  Sum1/1 -> M13/1  "M13"

== system V1/Non-sequential mixer/[P1] Control allocation/Subsystem16/Subsystem3 ==
  Bus Selector : BusSelector  OutputSignals=theta_4
  Bus Selector1 : BusSelector  OutputSignals=theta_4
  Gain : Gain  Gain=1/sqrt(2)
  Gain1 : Gain  Gain=1/sqrt(2)
  Product : Product
  Product1 : Product
  Sum : Sum  Inputs=|+-
  Sum1 : Sum  Inputs=|++
  Sum2 : Sum  Inputs=|+-
  Sum3 : Sum  Inputs=|--
  Trigonometric Function : Trigonometry  Operator=cos
  Trigonometric Function1 : Trigonometry
  M14 : Outport
  wires:
  Product/1 -> Sum1/1
  Sum/1 -> Product/1
  Sum2/1 -> Sum3/1
  Trigonometric Function/1 -> Product/2
  Bus Selector/1 -> Trigonometric Function/1  "<theta_4>"
  [hat_a] -> Sum2/1
  Gain/1 -> Sum/2
  Sum3/1 -> Gain1/1
  [hat_b_over_k] -> Sum3/2
  Gain1/1 -> Product1/1
  [hat_l] -> Gain/1
  Product1/1 -> Sum1/2
  Trigonometric Function1/1 -> Product1/2
  Bus Selector1/1 -> Trigonometric Function1/1  "<theta_4>"
  [Sensor] -> Bus Selector/1
  [Sensor] -> Bus Selector1/1
  Sum1/1 -> M14/1  "M14"
